simulink model "testMultitime"  (R2018a)
settings: Solver=VariableStepAuto  StartTime=0.0  StopTime=inf  RelTol=1e-3
values from neighbouring files (symbols this model uses):
  limit = generateRectangle(mapDim(1)-2,mapDim(2)-2)    [initialize.m]
  mode = 0    [initialize.m]
  scan_decoded = zeros(1081, 2)    [getHokuyoScan.m]
  sObs = nan(2, 3)    [initialize.m]
settings Model: Creator=alex  LastModifiedBy=hal

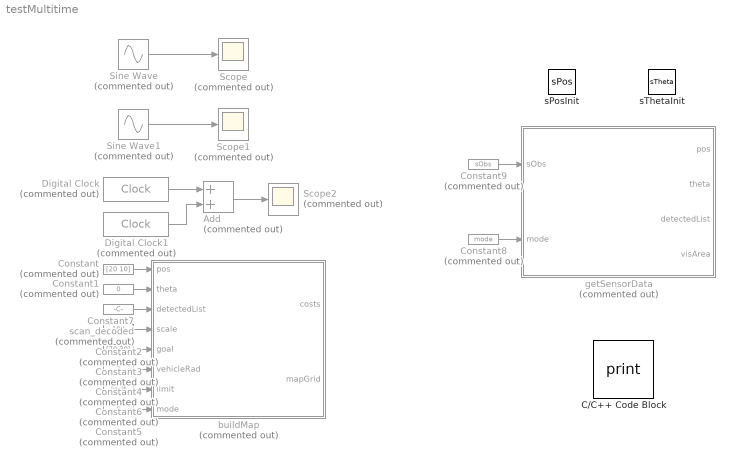
== system testMultitime ==
  Add : Sum  Commented=on
  C/C++ Code Block : S-Function  InitFcn=try, set_param(gcb,'FunctionName','print'), end  FunctionName=print  SFunctionDeploymentMode=off  EnableBusSupport=off  mask(S-Function Builder){}
      mask help: Simulink:masks:SFunctionBuilder_MD
      mask init:
      | val = [[.9  0.75 0.75 1 1 .9 .9 1]',[1 1 0.75 0.75 .9 .9 1 .9]'];try , sys = get_param(gcb,'SfunBuilderFcnName');if isempty(sys), sys = get_param(gcb,'FunctionName'); end,catch, sys = get_param(gcb,'FunctionName'); end
      settings: CopyFcn=set_param(gcbh,'LinkStatus','none')  PreSaveFcn=try, set_param(gcb,'FunctionName','print'), end  OpenFcn=sfunctionwizard(gcbh)
      mask Display: plot(val(:,1),val(:,2)),disp(sys), port_label('input',1,'u0'), port_label('output',1,'y0')
  Constant : Constant  Commented=on  Value=[20 10]  VectorParams1D=off
  Constant1 : Constant  Commented=on  Value=0  VectorParams1D=off
  Constant2 : Constant  Commented=on  Value=100  VectorParams1D=off
  Constant3 : Constant  Commented=on  Value=[70 30]  VectorParams1D=off
  Constant4 : Constant  Commented=on  Value=2  VectorParams1D=off
  Constant5 : Constant  Commented=on  Value=0  VectorParams1D=off
  Constant6 : Constant  Commented=on  Value=limit  VectorParams1D=off
  Constant7 : Constant  Commented=on  Value=scan_decoded  VectorParams1D=off
  Constant8 : Constant  Commented=on  Value=mode  VectorParams1D=off
  Constant9 : Constant  Commented=on  Value=sObs  VectorParams1D=off
  Digital Clock : DigitalClock  Commented=on  SampleTime=0.1
  Digital Clock1 : DigitalClock  Commented=on
  Scope : Scope  Commented=on
  Scope1 : Scope  Commented=on
  Scope2 : Scope  Commented=on
  Sine Wave : Sin  Commented=on  Frequency=20  SampleTime=0.1
  Sine Wave1 : Sin  Commented=on  SampleTime=1
  buildMap : MATLAB Function  Commented=on  TreatAsAtomicUnit=on
  getSensorData : MATLAB Function  Commented=on  TreatAsAtomicUnit=on  SystemSampleTime=0.1
  sPosInit : DataStoreMemory  DataStoreName=sPos  ReadBeforeWriteMsg=warning  WriteAfterWriteMsg=warning  WriteAfterReadMsg=warning  InitialValue=[10 10]  VectorParams1D=off  ShowAdditionalParam=off  OutDataTypeStr=double  Dimensions=[1 2]
  sThetaInit : DataStoreMemory  DataStoreName=sTheta  ReadBeforeWriteMsg=warning  WriteAfterWriteMsg=warning  WriteAfterReadMsg=warning  InitialValue=pi/2  ShowAdditionalParam=off  OutDataTypeStr=double  Dimensions=1
  wires:
  Sine Wave1/1 -> Scope1/1
  Sine Wave/1 -> Scope/1
  Digital Clock1/1 -> Add/2
  Digital Clock/1 -> Add/1
  Add/1 -> Scope2/1
  Constant/1 -> buildMap/1(pos)
  Constant1/1 -> buildMap/2(theta)
  Constant2/1 -> buildMap/4(scale)
  Constant3/1 -> buildMap/5(goal)
  Constant4/1 -> buildMap/6(vehicleRad)
  Constant5/1 -> buildMap/8(mode)
  Constant7/1 -> buildMap/3(detectedList)
  Constant6/1 -> buildMap/7(limit)
  Constant9/1 -> getSensorData/1(sObs)
  Constant8/1 -> getSensorData/2(mode)

== matlab function testMultitime/getSensorData ==
  data: sObs input; mode input; pos output; theta output; detectedList output; visArea output; sPos data_store_memory; sTheta data_store_memory
function [pos, theta, detectedList, visArea] = getSensorData(sObs, mode) 
    coder.extrinsic('serial', 'instrfind')   
    coder.extrinsic('tic')
    coder.extrinsic('toc')
    persistent t1
    if isempty(t1)
        t1 = tic;
    end
    time = toc(t1);
    t1 = tic;
    t2 = tic;
    fprintf('total calculation completed in %f seconds\n', time)
    fprintf('***************************************************\n');
    
    port_hokuyo = '/dev/ttyACM1';
    port_pozyx = '/dev/ttyUSB0';
    
    persistent COM_hokuyo COM_pozyx
    
    pos = [0 0];
    theta = 0;
    
    %% Real position and orientation 
    if mode == 0
%         if isempty(COM_pozyx)
%             if isempty(instrfind('Port', port_pozyx))
%                 COM_pozyx = serial(port_pozyx); 
%             else
%                 COM_pozyx = instrfind('Port', port_pozyx');
%             end
%             set(COM_pozyx, 'BaudRate', 115200)
%             set(COM_pozyx, 'Timeout', 10)
%             set(COM_pozyx, 'InputBufferSize', 128)
%             set(COM_pozyx, 'ReadAsyncMode', 'manual')
%             fclose(COM_pozyx);
%             fopen(COM_pozyx); 
%         end
%         
%         [pos, theta] = getPozyxData(COM_pozyx);
        pos = [20 10];
        theta = 0;
    end
    
    %% Simulation position and orientation 
    % starting position and orientation from simulink config
    global sPos sTheta   

    if mode == 1 
        % update simulation position and theta 
        pos = sPos;
        theta = sTheta;
    end
    
    %% Create vision area visual object 
    if mode == 1 
        % visArea opening angle above/below horizontal and leg length 
        coneAngle = pi/2.5;
        coneDepth = 100;
        
        % 4 points to make visArea in polar rotated to current theta  
        t = [0 coneAngle -coneAngle 0] + theta;
        r = [0 coneDepth coneDepth 0];
        
        % convert to cartesian, z column for compatability with built-in trig 
        [x, y] = pol2cart(t, r);
        z = zeros(1,4);
        
        % list format and translate to current pos 
        visArea = rot90(vertcat(z,y,x),3);
        visArea(:,1) = visArea(:,1) + pos(1);
        visArea(:,2) = visArea(:,2) + pos(2);
    else 
        lineLength = 8;
        t = [-3*pi/4 0 0 3*pi/4] + theta;
        r = [lineLength 0 0 lineLength];
        
        [x, y] = pol2cart(t, r);
        z = zeros(1,4);
        
        visArea = rot90(vertcat(z,y,x),3);
        visArea(:,1) = visArea(:,1) + pos(1);
        visArea(:,2) = visArea(:,2) + pos(2);
        
    end
    
    %% Real obstacle detection
    % lidar scan list from Hokuyo UTM-30LX
    nPoints = 1081;
    detectedList = repmat([nan nan], nPoints, 1); 
    if mode == 0
        if isempty(COM_hokuyo)
            if isempty(instrfind('Port', port_hokuyo))
                COM_hokuyo = serial(port_hokuyo); 
            else
                COM_hokuyo = instrfind('Port', port_hokuyo');
            end
            set(COM_hokuyo, 'Timeout', 10)
            fclose(COM_hokuyo);
            fopen(COM_hokuyo); 
        end
        disp('d1')
        detectedList = getHokuyoScan(COM_hokuyo);
        disp('d2')
    end
    
    %% Simulation obstacle detection 
    if mode == 1
        % get detected vector 
        sObsList = reshape(permute(sObs,[2,1,3]),size(sObs,2),[])';
        detected = detectRotated(sObsList, visArea);

        % list obstacles that are detected 
        if any(detected)
            detectedListTemp2 = repmat([nan nan], nPoints, 1); 

            sObsListX = sObsList(:,1);
            sObsListY = sObsList(:,2);
            detectedListX = sObsListX(detected==1);
            detectedListY = sObsListY(detected==1);
            detectedListTemp1 = horzcat(detectedListX, detectedListY);
            detectedListTemp2(:) = vertcat(detectedListTemp1,...
                repmat([nan nan], nPoints-size(detectedListTemp1, 1), 1));
            detectedList = detectedListTemp2;
        end
    end
    
    time = toc(t2);
    fprintf('getSensorData completed in %f seconds\n', time)
end

== matlab function testMultitime/buildMap ==
  data: pos input; costs output size=[1 ((mapDim(1)-1)*(mapDim(2)-1)*3)+9]; theta input; detectedList input; scale input; goal input; vehicleRad input; limit input; mode input; mapGrid output size=[mapDim(2)-1 mapDim(1)-1]
function [costs, mapGrid] = buildMap(pos, theta, detectedList, scale, goal, vehicleRad,...
                                        limit, mode)
    coder.extrinsic('tic')
    coder.extrinsic('toc')
    coder.varsize('roundedLimitUnique');
    
    t1 = tic;
    
    mapDim = [80 40]; %[40 20]; % must be equalivant in initialize.m
    
    persistent mapGridP 
    if isempty(mapGridP)
        mapGridP = zeros(mapDim(2)-1, mapDim(1)-1);
    end
    
    %% Reduce resolution of raw lidar data by 100
    compressed = nan;
    if mode == 0
        compressed = [detectedList(:,1) detectedList(:,2) / 100];
    end
        
    %% Orient polar list and convert to certesian 
    orientCart = nan;
    if mode == 0
        compressed(:,1) = compressed(:,1) + theta - pi/2;
        [detX, detY] = pol2cart(compressed(:,1), compressed(:,2));
        orientCart = [detX detY];
    end
    
    %% Translate cartesian list, round 
    offset = 1.2; % MOVE to simulink level: measurement lidar to midpoint in decimeter 
    
    transCart = nan;
    if mode == 0
        transCart = orientCart;
        transCart(:,1) = transCart(:,1) + pos(1) + offset*cos(theta); 
        transCart(:,2) = transCart(:,2) + pos(2) + offset*sin(theta);
    end
    
    %% Round list and eliminate duplicate points
    roundedUnique = nan;
    if mode == 0
        roundTransCart = round(transCart);
        roundedUnique = unique(roundTransCart, 'rows');
    end
        
    %% Sim data is already rounded and has no duplicates  
    if mode == 1
        roundedUnique = detectedList;
    end

    %% Add 2D map boundary to obstacle data 
    roundedLimitUnique = [limit(:,1:2); roundedUnique(:,1:2)]; 
    
    %% Eliminate points outside limit and Nan entries 
    roundedLimitUnique(isnan(roundedLimitUnique(:,1)), :) = [];
    roundedLimitUnique(roundedLimitUnique(:, 1) <= 0, :) = [];
    roundedLimitUnique(roundedLimitUnique(:, 1) > mapDim(1)-1, :) = [];
    roundedLimitUnique(roundedLimitUnique(:, 2) <= 0, :) = [];
    roundedLimitUnique(roundedLimitUnique(:, 2) > mapDim(2)-1, :) = [];
    
    %% Convert list to grid 
    limitGrid = list2grid(roundedLimitUnique(:,1), roundedLimitUnique(:,2), mapDim(1)-1, mapDim(2)-1);

    %% Inflate points 
    t2 = tic;
    inflated = inflate2(limitGrid, vehicleRad);
    time = toc(t2);
    fprintf('inflation completed in %f seconds\n', time)

    %% Persist grid and average with new 
    if mode == 0
        alpha = 0.8; beta = 0.2;
    else
        alpha = 0.99; beta = 0.01;
    end
    mapGridP = alpha*mapGridP + beta*inflated;
    mapGrid = mapGridP;
    
    %% Convert probability grid to list for d*
    mapList = grid2list(mapGrid);
    
    % convert into 1-by vector: size pos goal mapList1:end
    costsTemp = vertcat([numel(mapList)/3 0 0], [pos 0], [goal 0], mapList);
    costs = reshape(costsTemp.',1,numel(costsTemp));
    
    time = toc(t1);
    fprintf('buildMap completed in %f seconds\n', time)
    tic
    
end
